simulink model "doc_agc_plot_step_size"  (R2014a)
settings: Solver=FixedStepDiscrete  StartTime=0.0  StopTime=2e3  RelTol=1e-3
libraries: commrfcorlib x2, commdigbbndpm3 x1, commrandsrc2 x1
settings Model: Creator=The MathWorks Inc.
settings DebuggingCC: UnderspecifiedInitializationDetection=Classic  StateNameClashWarn=warning

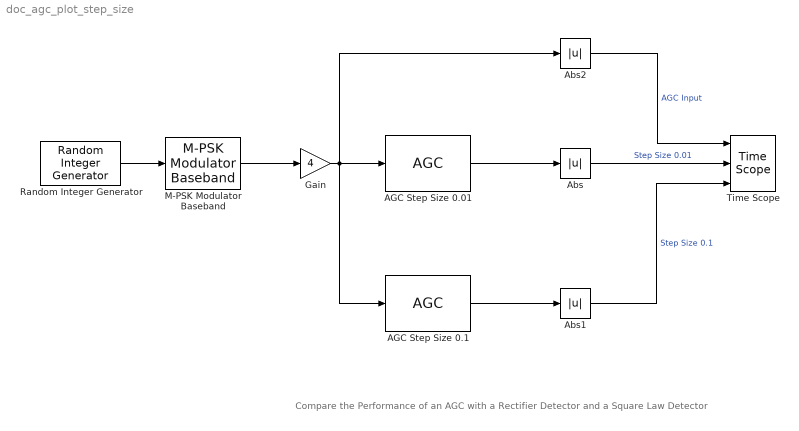
== system doc_agc_plot_step_size ==
  note: Compare the Performance of an AGC with a Rectifier Detector and a Square Law Detector
  "AGC Step Size 0.01 " : commrfcorlib/AGC  SimulateUsing=Code generation  DetectorMethod=Rectifier  LoopMethod=Linear  UpdatePeriod=10  StepSize=0.01  MaximumGain=30  GainOutputPort=off
  "AGC Step Size 0.1 " : commrfcorlib/AGC  SimulateUsing=Code generation  DetectorMethod=Rectifier  LoopMethod=Linear  UpdatePeriod=10  StepSize=0.1  MaximumGain=30  GainOutputPort=off
  Abs : Abs
  Abs1 : Abs
  Abs2 : Abs
  Gain : Gain  Gain=4
  M-PSK Modulator Baseband : commdigbbndpm3/M-PSK Modulator Baseband  M=4  InType=Integer  Enc=Gray  Mapping=[0:7]  Ph=pi/4  outDtype=double  outWordLen=16  outUDDataType=sfix(16)  outFracLenMode=Best precision  outFracLen=15
  Random Integer Generator : commrandsrc2/Random Integer Generator  mul=4  seed=37  Ts=1  frameBased=on  sampPerFrame=1000  orient=off  outDataType=double
  Time Scope : TimeScope  NumInputPorts=3  DefaultConfigurationName=spbscopes.TimeScopeBlockCfg
  wires:
  Random Integer Generator/1 -> M-PSK Modulator Baseband/1
  M-PSK Modulator Baseband/1 -> Gain/1
  "AGC Step Size 0.01 "/1 -> Abs/1
  Gain/1 -> Abs2/1, "AGC Step Size 0.1 "/1, "AGC Step Size 0.01 "/1
  "AGC Step Size 0.1 "/1 -> Abs1/1
  Abs/1 -> Time Scope/2  "Step Size 0.01"
  Abs1/1 -> Time Scope/3  "Step Size 0.1"
  Abs2/1 -> Time Scope/1  "AGC Input"
